simulink model "ass3_freq_estimation"  (R2021a)
settings: Solver=VariableStepAuto  StartTime=0.0  StopTime=1500  RelTol=1e-3
settings Model: Creator=valerio  LastModifiedBy=valerio

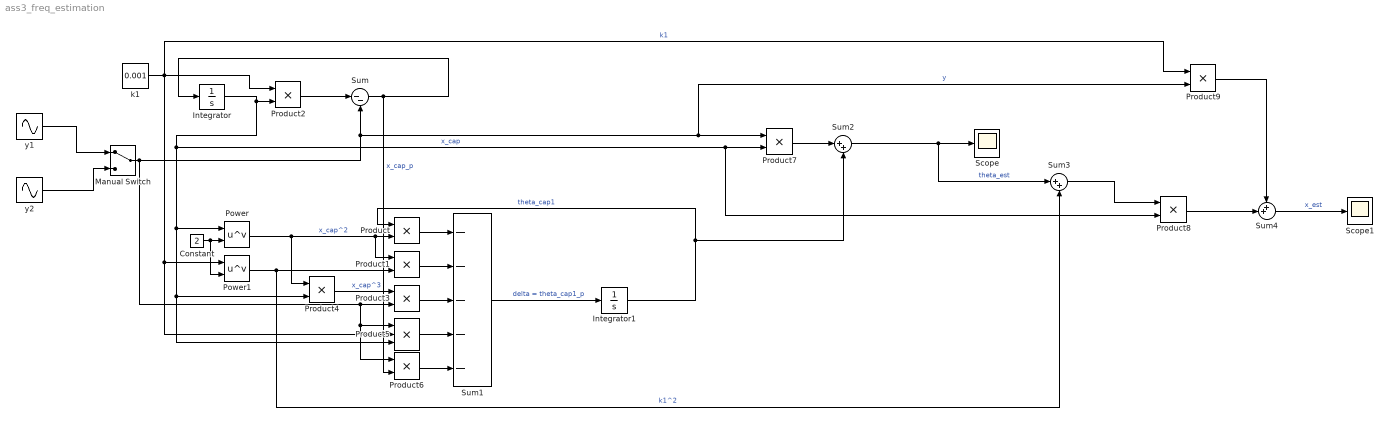
== system ass3_freq_estimation ==
  Constant : Constant  Value=2
  Integrator : Integrator
  Integrator1 : Integrator
  Manual Switch : ManualSwitch
  Power : Math  Operator=pow  SaturateOnIntegerOverflow=on
  Power1 : Math  Operator=pow  SaturateOnIntegerOverflow=on
  Product{,1..4,6..9} (9 alike) : Product
  Product5 : Product  Inputs=3
  Scope : Scope
  Scope1 : Scope
  Sum : Sum  Inputs=|--
  Sum1 : Sum  Inputs=-----
  Sum2 : Sum  Inputs=|++
  Sum3 : Sum  Inputs=|++
  Sum4 : Sum  Inputs=++|
  k1 : Constant  Value=0.001
  y1 : Sin  Frequency=100  SampleTime=0
  y2 : Sin  SampleTime=0
  wires:
  y1/1 -> Manual Switch/1
  y2/1 -> Manual Switch/2
  Integrator/1 -> Product2/2, Product8/2, Product7/2, Product5/3, Product4/2, Power/1  "x_cap"
  Manual Switch/1 -> Product6/1, Product5/1, Product3/2, Sum/2, Product9/2, Product7/1  "y"
  Sum/1 -> Product6/2, Integrator/1  "x_cap_p"
  Sum1/1 -> Integrator1/1  "delta = theta_cap1_p"
  Integrator1/1 -> Sum2/2, Product/1  "theta_cap1"
  Power/1 -> Product4/1, Product1/1, Product/2  "x_cap^2"
  Constant/1 -> Power1/2, Power/2
  Product/1 -> Sum1/1
  Product2/1 -> Sum/1
  k1/1 -> Product5/2, Power1/1, Product9/1, Product2/1  "k1"
  Power1/1 -> Sum3/2, Product1/2  "k1^2"
  Product1/1 -> Sum1/2
  Product3/1 -> Sum1/3
  Product4/1 -> Product3/1  "x_cap^3"
  Product5/1 -> Sum1/4
  Product6/1 -> Sum1/5
  Product7/1 -> Sum2/1
  Sum2/1 -> Sum3/1, Scope/1  "theta_est"
  Sum3/1 -> Product8/1
  Product8/1 -> Sum4/2
  Product9/1 -> Sum4/1
  Sum4/1 -> Scope1/1  "x_est"
